simulink model "Reg_disc"  (R2023b)
settings: Solver=FixedStepDiscrete  StartTime=0.0  StopTime=10.0  RelTol=1e-3
settings Model: Creator=ycheb  LastModifiedBy=ycheb

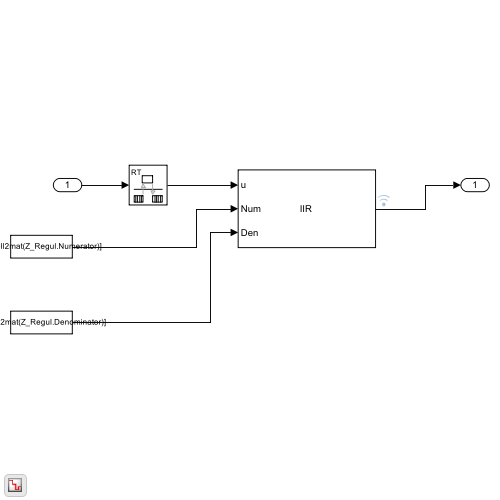
[thumbnail: Simulink's stored preview of the top-level diagram]
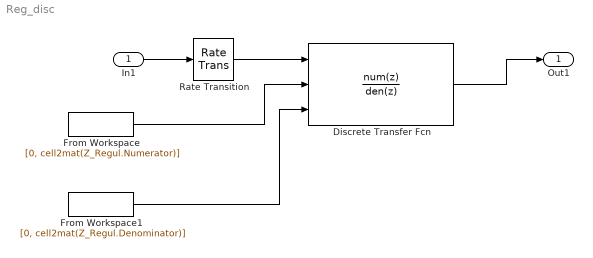
== system Reg_disc ==
  In1 : Inport
  Discrete Transfer Fcn : DiscreteTransferFcn  NumeratorSource=Input port  Numerator=[433.4046 -866.3778 432.9733]  DenominatorSource=Input port  Denominator=[1 -1.7828 0.7828]  a0EqualsOne=on
      settings: InputPortMap=u0,p1,p3
  From Workspace : FromWorkspace  VariableName=[0, cell2mat(Z_Regul.Numerator)]  SampleTime=-1
  From Workspace1 : FromWorkspace  VariableName=[0, cell2mat(Z_Regul.Denominator)]  SampleTime=-1
  Rate Transition : RateTransition  OutPortSampleTime=1e-4
  Out1 : Outport
  wires:
  In1/1 -> Rate Transition/1
  Rate Transition/1 -> Discrete Transfer Fcn/1
  Discrete Transfer Fcn/1 -> Out1/1
  From Workspace/1 -> Discrete Transfer Fcn/2
  From Workspace1/1 -> Discrete Transfer Fcn/3
